simulink model "daq2_sim_org"  (Simulink 10.0)
settings: Solver=ode45  StartTime=0.0  StopTime=Inf  RelTol=1e-3  EnableMultiTasking=on
libraries: dspsrcs4 x2
settings Model: Creator=ACozma  LastModifiedBy=bhisma
settings DataIOCC: LimitDataPoints=on
settings DebuggingCC: SolverPrmCheckMsg=warning  AllowSymbolicDim=off
settings GRTTargetCC: GeneratePreprocessorConditionals=Disable all  CombineOutputUpdateFcns=on  GRTInterface=off
settings ConfigComp: CovExternalEMLEnable=off  CovSFcnEnable=off

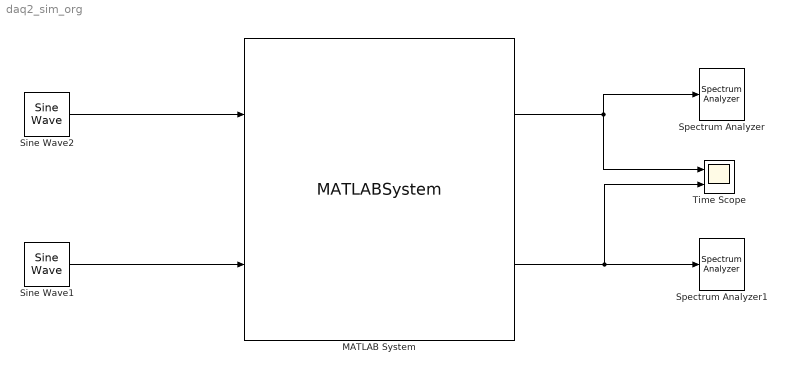
== system daq2_sim_org ==
  MATLAB System : MATLABSystem  DialogController=sysobjdialog.BlockDynDialog  System=iio_sys_obj  ip_address=10.50.1.113  dev_name=daq2  in_ch_no=2  in_ch_size=8192*128  out_ch_no=2  out_ch_size=8192*128  SimulateUsing=Interpreted execution
      mask Type: iio_sys_obj
      mask Display:
      | disp('daq2');
      | port_label('input',1,'DATA_IN1');
      | port_label('input',2,'DATA_IN2');
      | port_label('output',1,'DATA_OUT1');
      | port_label('output',2,'DATA_OUT2');
  Sine Wave1 : dspsrcs4/Sine Wave  Amplitude=8192  Frequency=20e6  Phase=pi/2  SampleMode=Discrete  OutComplex=Real  CompMethod=Differential  TableSize=Speed  SampleTime=1/1000000000  SamplesPerFrame=8192*128  ResetState=Restart at time zero  OutputFrames=on  dataType=double  wordLen=16  udDataType=sfix(16)  fracBitsMode=Best precision  numFracBits=15  OutDataTypeStr=double  LastOutDataTypeStr=double
  Sine Wave2 : dspsrcs4/Sine Wave  Amplitude=8192  Frequency=20e6  Phase=0  SampleMode=Discrete  OutComplex=Real  CompMethod=Differential  TableSize=Speed  SampleTime=1/1000000000  SamplesPerFrame=8192*128  ResetState=Restart at time zero  OutputFrames=on  dataType=double  wordLen=16  udDataType=sfix(16)  fracBitsMode=Best precision  numFracBits=15  OutDataTypeStr=double  LastOutDataTypeStr=double
  Spectrum Analyzer : SpectrumAnalyzer
  Spectrum Analyzer1 : SpectrumAnalyzer
  Time Scope : Scope  NumInputPorts=2
  wires:
  MATLAB System/1 -> Spectrum Analyzer/1, Time Scope/1
  Sine Wave2/1 -> MATLAB System/1
  Sine Wave1/1 -> MATLAB System/2
  MATLAB System/2 -> Spectrum Analyzer1/1, Time Scope/2
